simulink model "Three_phase_DAB_converter_2_"  (R2025b)
settings: Solver=VariableStepAuto  StartTime=0.0  StopTime=1  RelTol=1e-3
undefined symbols (not defined in the file): Ion, Lithium
libraries: eeRmsMeasurement x4, spsBatteryLib x2, spsUniversalBridgeLib x2, spsSeriesRLCBranchLib x2, eeGeneralControl x2, spsPower3phInstantaneousLib x2, spsThreePhaseVIMeasurementLib x2, spsThreePhaseSeriesRLCBranchLib x1, spsThreePhaseTransformerTwoWindingsLib x1, sps_lib x1
settings Model: Creator=91637  LastModifiedBy=DELL

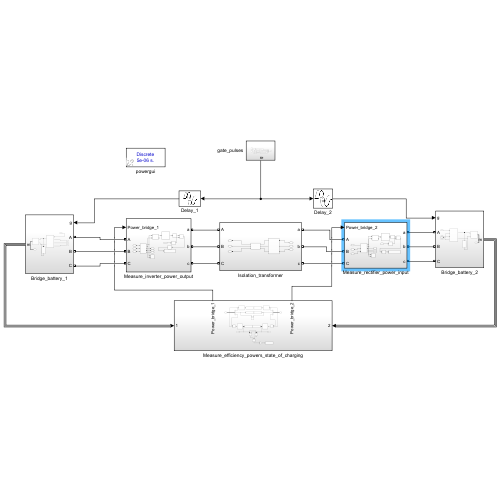
[thumbnail: Simulink's stored preview of the top-level diagram]
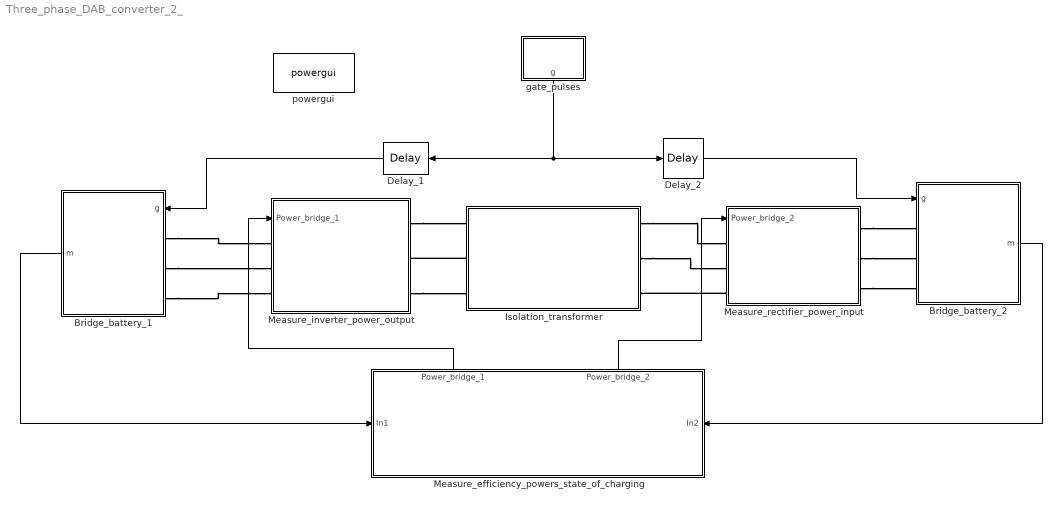
== system Three_phase_DAB_converter_2_ ==
  Bridge_battery_1 : Subsystem
  Bridge_battery_2 : Subsystem
  Delay_1 : TransportDelay  DelayTime=5e-6  BufferSize=1e5
  Delay_2 : TransportDelay  DelayTime=0
  Isolation_transformer : Subsystem
  Measure_efficiency_powers_state_of_charging : Subsystem
      settings: PortSchema="{\"entries\":[{\"content\":{\"sides\":[{\"content\":{\"connectorIds\":[\"In1\"]},\"type\":\"ConnectorPlacement.EquallySpacedRectSide\",\"uuid\":\"727947a8-7189-4754-ba39-ed4545685221\"},{\"content\":{\"connectorIds\":[\"In2\"],\"side\":\"RIGHT\"},\"type\":\"ConnectorPlacement.EquallySpacedRectSide\",\"uuid\":\"4f4ff040-aa02-42b0-ba60-9cf53e88cf93\"},{\"content\":{\"connectorIds\":[\"Out1\",\"Out2\"],\"side\":\"TOP\"},\"type\":\"ConnectorPlacement.EquallySpacedRectSide\",\"uuid\":\"ace19928-1506-4de9-a11d-c8770fc65bb2\"}]},\"type\":\"ConnectorPlacement.EquallySpacedConnector\",\"uuid\":\"7c6c4745-ab83-4df3-9031-3474db267f64\"}],\"packageUris\":[\"http://schema.mathworks.com/mf0/Connector/R2020b\"],\"version\":\"1.0\"}"
  Measure_inverter_power_output : Subsystem
  Measure_rectifier_power_input : Subsystem
  gate_pulses : Subsystem
  powergui : sps_lib/powergui  Priority=1  SimulationMode=Discrete  SampleTime=5e-6  frequency=60  Iterations=50  frequencyindice=0  Pbase=100e6  ErrMax=1e-4  UnitsV=kV  UnitsW=MW  buscounter=0  FunctionMessages=off  echomessages=off  EnableUseOfTLC=off  CurrentSourceSwitches=off  DisableSnubberDevices=off  DisableRonSwitches=off  DisableVfSwitches=off  DisplayEquations=off  AutomaticDiscreteSolvers=off  SolverType=Tustin/Backward Euler (TBE)  Interpol=off  ExternalGateDelay=off  methode=off  Ts=100  x0status=blocks  SPID=on  SwTol=0  HookPort=off  NonlinearTolerance=1e-4  nMaxIteration=100  ContinueOnMaxIteration=off  RestoreLinks=warning  ResistiveCurrentMeasurement=off  Frange=[0:2:500]  Ylog=off  Xlog=on  ShowGrid=off  save=off  variable=ZData  structure=0  ZoomFFT=off  StartTime=0.0  cycles=1  DisplayStyle=1  fundamental=60  FreqAxis=off  MaxFrequency=1000  frequencyindicesteady=1  RmsSteady=1  display=off
  wires:
  Bridge_battery_2/1(m) -> Measure_efficiency_powers_state_of_charging/2(In2)
  gate_pulses/1(g) -> Delay_2/1, Delay_1/1
  Bridge_battery_1/1(m) -> Measure_efficiency_powers_state_of_charging/1(In1)
  Measure_efficiency_powers_state_of_charging/2(Power_bridge_2) -> Measure_rectifier_power_input/1(Power_bridge_2)
  Measure_efficiency_powers_state_of_charging/1(Power_bridge_1) -> Measure_inverter_power_output/1(Power_bridge_1)
  Delay_1/1 -> Bridge_battery_1/1(g)
  Delay_2/1 -> Bridge_battery_2/1(g)
  connections:
  Isolation_transformer/RConn1 -- Measure_rectifier_power_input/LConn1
  Measure_rectifier_power_input/RConn1 -- Bridge_battery_2/LConn1
  Isolation_transformer/RConn2 -- Measure_rectifier_power_input/LConn2
  Measure_rectifier_power_input/RConn2 -- Bridge_battery_2/LConn2
  Measure_rectifier_power_input/LConn3 -- Isolation_transformer/RConn3
  Measure_rectifier_power_input/RConn3 -- Bridge_battery_2/LConn3
  Measure_inverter_power_output/RConn1 -- Isolation_transformer/LConn1
  Bridge_battery_1/LConn1 -- Measure_inverter_power_output/LConn1
  Isolation_transformer/LConn2 -- Measure_inverter_power_output/RConn2
  Bridge_battery_1/LConn2 -- Measure_inverter_power_output/LConn2
  Measure_inverter_power_output/RConn3 -- Isolation_transformer/LConn3
  Bridge_battery_1/LConn3 -- Measure_inverter_power_output/LConn3

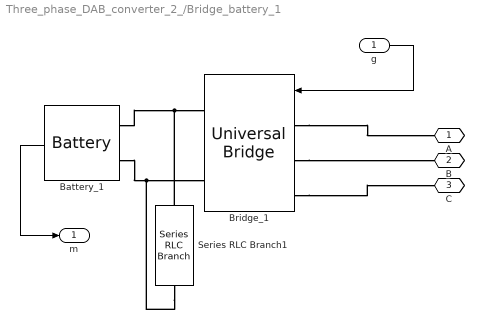
== system Three_phase_DAB_converter_2_/Bridge_battery_1 ==
  g : Inport
  Battery_1 : spsBatteryLib/Battery  BatType=Lithium-Ion  NomV=48  NomQ=20  SOC=80  Batt_Tr=0.01  PresetModel=on  MaxQ=20  MinV=36  FullV=55.8714  Dis_rate=8.6957  R=0.024  Normal_OP=18.087  expZone="[51.8585     0.982609]"
  Bridge_1 : spsUniversalBridgeLib/Universal Bridge  Arms=3  SnubberResistance=1e5  SnubberCapacitance=inf  Device=MOSFET / Diodes  Ron=1e-3  Lon=0  ForwardVoltages="[  0  0  ]"  ForwardVoltage=0  GTOparameters=[ 10e-6 , 20e-6 ]  IGBTparameters=[ 1e-6 , 2e-6 ]  Measurements=None  Measurements_2=None  converterType=Rectifier
      link override Status: GotoTag=T49_4813_4131163465740
  Series RLC Branch1 : spsSeriesRLCBranchLib/Series RLC Branch  LConnTagsString=__new0  RConnTagsString=__new0  BranchType=RC  Resistance=1000  Inductance=1e-3  SetiL0=off  InitialCurrent=0  Capacitance=1000e-6  Setx0=off  InitialVoltage=0  Measurements=None
  A : PMIOPort  Side=Left
  B : PMIOPort  Port=2  Side=Left
  C : PMIOPort  Port=3  Side=Left
  m : Outport
  wires:
  g/1 -> Bridge_1/1
  Battery_1/1 -> m/1
  connections:
  Bridge_1/LConn1 -- A/RConn1
  Battery_1/LConn2 -- Series RLC Branch1/RConn1 -- Bridge_1/RConn2
  Bridge_1/LConn3 -- C/RConn1
  Battery_1/LConn1 -- Series RLC Branch1/LConn1 -- Bridge_1/RConn1
  Bridge_1/LConn2 -- B/RConn1

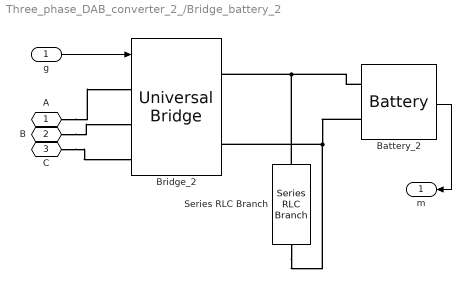
== system Three_phase_DAB_converter_2_/Bridge_battery_2 ==
  g : Inport
  Battery_2 : spsBatteryLib/Battery  BatType=Lithium-Ion  NomV=44  NomQ=20  SOC=40  Batt_Tr=0.01  PresetModel=on  MaxQ=20  MinV=33  FullV=51.2154  Dis_rate=8.6957  R=0.022  Normal_OP=18.087  expZone="[47.537     0.982609]"
  Bridge_2 : spsUniversalBridgeLib/Universal Bridge  Arms=3  SnubberResistance=1e5  SnubberCapacitance=inf  Device=MOSFET / Diodes  Ron=1e-3  Lon=0  ForwardVoltages="[  0  0  ]"  ForwardVoltage=0  GTOparameters=[ 10e-6 , 20e-6 ]  IGBTparameters=[ 1e-6 , 2e-6 ]  Measurements=None  Measurements_2=None  converterType=Rectifier
  Series RLC Branch : spsSeriesRLCBranchLib/Series RLC Branch  LConnTagsString=__new0  RConnTagsString=__new0  BranchType=RC  Resistance=1000  Inductance=1e-3  SetiL0=off  InitialCurrent=0  Capacitance=1000e-6  Setx0=off  InitialVoltage=0  Measurements=None
  A : PMIOPort  Side=Left
  B : PMIOPort  Port=2  Side=Left
  C : PMIOPort  Port=3  Side=Left
  m : Outport
  wires:
  g/1 -> Bridge_2/1
  Battery_2/1 -> m/1
  connections:
  C/RConn1 -- Bridge_2/LConn3
  Battery_2/LConn2 -- Series RLC Branch/RConn1 -- Bridge_2/RConn2
  B/RConn1 -- Bridge_2/LConn2
  Battery_2/LConn1 -- Bridge_2/RConn1 -- Series RLC Branch/LConn1
  A/RConn1 -- Bridge_2/LConn1

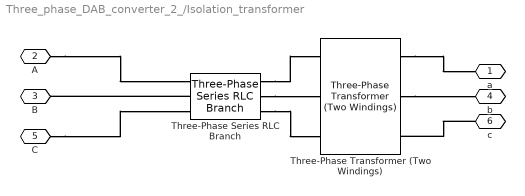
== system Three_phase_DAB_converter_2_/Isolation_transformer ==
  Three-Phase Series RLC Branch : spsThreePhaseSeriesRLCBranchLib/Three-Phase Series RLC Branch  LConnTagsString=A|B|C  RConnTagsString=A|B|C  BranchType=RL  Resistance=1e-2  Inductance=40e-6  Capacitance=1e-6  Measurements=None
  Three-Phase Transformer (Two Windings) : spsThreePhaseTransformerTwoWindingsLib/Three-Phase Transformer (Two Windings)  Winding1Connection=Yg  Winding2Connection=Yg  CoreType=Three single-phase transformers  SetSaturation=off  Hysteresis=off  DataFile='hysteresis'  SetInitialFlux=off  Measurements=None  UNITS=pu  NominalPower=[ 1e3 , 1e4 ]  Winding1=[230 0.003 0.01]  Winding2=[230 0.003 0.01]  Rm=500  Lm=200  L0=0.49999  Saturation=[0 0;0.0024 1.2;1 1.52]  InitialFluxes=[0.80001 -0.80001 0.7]  BreakLoop=off  DiscreteSolver=Trapezoidal iterative  DataType=off  TransfoNumber=1
  a : PMIOPort  Side=Right
  A : PMIOPort  Port=2  Side=Left
  B : PMIOPort  Port=3  Side=Left
  b : PMIOPort  Port=4  Side=Right
  C : PMIOPort  Port=5  Side=Left
  c : PMIOPort  Port=6  Side=Right
  connections:
  Three-Phase Series RLC Branch/RConn3 -- Three-Phase Transformer (Two Windings)/LConn3
  Three-Phase Transformer (Two Windings)/RConn1 -- a/RConn1
  c/RConn1 -- Three-Phase Transformer (Two Windings)/RConn3
  Three-Phase Transformer (Two Windings)/RConn2 -- b/RConn1
  Three-Phase Series RLC Branch/RConn1 -- Three-Phase Transformer (Two Windings)/LConn1
  A/RConn1 -- Three-Phase Series RLC Branch/LConn1
  Three-Phase Series RLC Branch/LConn2 -- B/RConn1
  Three-Phase Series RLC Branch/RConn2 -- Three-Phase Transformer (Two Windings)/LConn2
  C/RConn1 -- Three-Phase Series RLC Branch/LConn3

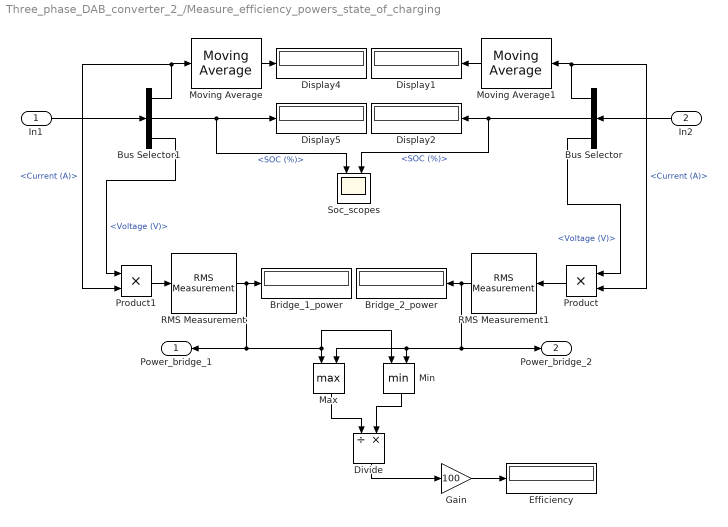
== system Three_phase_DAB_converter_2_/Measure_efficiency_powers_state_of_charging ==
  In1 : Inport
  In2 : Inport  Port=2
  Bridge_1_power : Display
  Bridge_2_power : Display
  Bus Selector : BusSelector  OutputSignals=Current (A),SOC (%),Voltage (V)
  Bus Selector1 : BusSelector  OutputSignals=Current (A),SOC (%),Voltage (V)
  Display{1..2,4..5} (4 alike) : Display
  Divide : Product  Inputs=/*
  Efficiency : Display
  Gain : Gain  Gain=100
  Max : MinMax  Function=max  Inputs=2
  Min : MinMax  Inputs=2
  Moving Average : eeGeneralControl/Moving Average  VariantControl=Variant1  LabelModeActiveChoice=Discrete  f=50  x0=0  BufferSize=8192  Ts=-1
      settings: LibrarySourceBlock=ee_sl_lib/General Control/Moving Average
  Moving Average1 : eeGeneralControl/Moving Average  VariantControl=Variant1  LabelModeActiveChoice=Discrete  f=50  x0=0  BufferSize=8192  Ts=-1
      settings: LibrarySourceBlock=ee_sl_lib/General Control/Moving Average
  Product : Product
  Product1 : Product
  RMS Measurement : eeRmsMeasurement/RMS Measurement  LabelModeActiveChoice=Total  F=60  SpecifyHarmonics=off  K=[0 1 2]  Ts=0
      settings: LibrarySourceBlock=|
      | ee_sl_lib/Measurements/RMS
      | Measurement
  RMS Measurement1 : eeRmsMeasurement/RMS Measurement  LabelModeActiveChoice=Total  F=60  SpecifyHarmonics=off  K=[0 1 2]  Ts=0
      settings: LibrarySourceBlock=|
      | ee_sl_lib/Measurements/RMS
      | Measurement
  Soc_scopes : Scope  NumInputPorts=2
      settings: ActiveDisplayYMinimum=80.6573374913129  ActiveDisplayYMaximum=80.660364899071055  DataLoggingVariableName=ScopeData2
  Power_bridge_1 : Outport  VectorParamsAs1DForOutWhenUnconnected=off
  Power_bridge_2 : Outport  Port=2
  wires:
  Product1/1 -> RMS Measurement/1
  Bus Selector1/1 -> Product1/2, Moving Average/1  "<Current (A)>"
  RMS Measurement1/1 -> Min/2, Max/2, Power_bridge_2/1, Bridge_2_power/1
  Bus Selector/1 -> Moving Average1/1, Product/2  "<Current (A)>"
  Moving Average1/1 -> Display1/1
  Bus Selector1/2 -> Soc_scopes/1, Display5/1  "<SOC (%)>"
  Bus Selector1/3 -> Product1/1  "<Voltage (V)>"
  Bus Selector/2 -> Soc_scopes/2, Display2/1  "<SOC (%)>"
  Moving Average/1 -> Display4/1
  In1/1 -> Bus Selector1/1
  Bus Selector/3 -> Product/1  "<Voltage (V)>"
  Product/1 -> RMS Measurement1/1
  RMS Measurement/1 -> Min/1, Max/1, Power_bridge_1/1, Bridge_1_power/1
  In2/1 -> Bus Selector/1
  Divide/1 -> Gain/1
  Gain/1 -> Efficiency/1
  Max/1 -> Divide/1
  Min/1 -> Divide/2

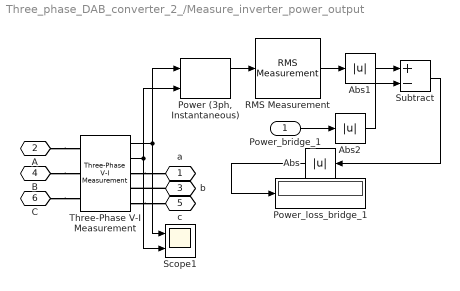
== system Three_phase_DAB_converter_2_/Measure_inverter_power_output ==
  Power_bridge_1 : Inport
  Abs : Abs  SaturateOnIntegerOverflow=off
  Abs1 : Abs  SaturateOnIntegerOverflow=off
  Abs2 : Abs  SaturateOnIntegerOverflow=off
  "Power (3ph, Instantaneous)" : spsPower3phInstantaneousLib/Power (3ph, Instantaneous)
  Power_loss_bridge_1 : Display
  RMS Measurement : eeRmsMeasurement/RMS Measurement  LabelModeActiveChoice=Total  F=60  SpecifyHarmonics=off  K=[0 1 2]  Ts=0
      settings: LibrarySourceBlock=|
      | ee_sl_lib/Measurements/RMS
      | Measurement
  Scope1 : Scope  NumInputPorts=2
      settings: ActiveDisplayYMinimum=-87.331585407459983  ActiveDisplayYMaximum=86.18489489271434
  Subtract : Sum  Inputs=+-
  Three-Phase V-I Measurement : spsThreePhaseVIMeasurementLib/Three-Phase V-I Measurement  VoltageMeasurement=phase-to-ground  SetLabelV=off  LabelV=Vabc  Vpu=off  VpuLL=off  CurrentMeasurement=yes  SetLabelI=off  LabelI=Iabc  Ipu=off  Pbase=100e6  Vbase=500e3  OutputType=Complex  PhasorSimulation=off  PSBequivalent=0
  a : PMIOPort  Side=Right
  A : PMIOPort  Port=2  Side=Left
  b : PMIOPort  Port=3  Side=Right
  B : PMIOPort  Port=4  Side=Left
  c : PMIOPort  Port=5  Side=Right
  C : PMIOPort  Port=6  Side=Left
  wires:
  Three-Phase V-I Measurement/1 -> "Power (3ph, Instantaneous)"/1, Scope1/1
  Three-Phase V-I Measurement/2 -> "Power (3ph, Instantaneous)"/2, Scope1/2
  "Power (3ph, Instantaneous)"/1 -> RMS Measurement/1
  Abs/1 -> Power_loss_bridge_1/1
  Subtract/1 -> Abs/1
  Power_bridge_1/1 -> Abs2/1
  RMS Measurement/1 -> Abs1/1
  Abs1/1 -> Subtract/1
  Abs2/1 -> Subtract/2
  connections:
  b/RConn1 -- Three-Phase V-I Measurement/RConn2
  Three-Phase V-I Measurement/RConn3 -- c/RConn1
  Three-Phase V-I Measurement/RConn1 -- a/RConn1
  A/RConn1 -- Three-Phase V-I Measurement/LConn1
  B/RConn1 -- Three-Phase V-I Measurement/LConn2
  C/RConn1 -- Three-Phase V-I Measurement/LConn3

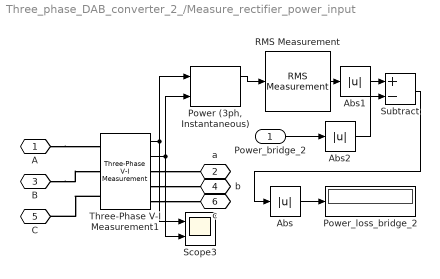
== system Three_phase_DAB_converter_2_/Measure_rectifier_power_input ==
  Power_bridge_2 : Inport
  Abs : Abs  SaturateOnIntegerOverflow=off
  Abs1 : Abs  SaturateOnIntegerOverflow=off
  Abs2 : Abs  SaturateOnIntegerOverflow=off
  "Power (3ph, Instantaneous)" : spsPower3phInstantaneousLib/Power (3ph, Instantaneous)
  Power_loss_bridge_2 : Display
  RMS Measurement : eeRmsMeasurement/RMS Measurement  LabelModeActiveChoice=Total  F=60  SpecifyHarmonics=off  K=[0 1 2]  Ts=0
      settings: LibrarySourceBlock=|
      | ee_sl_lib/Measurements/RMS
      | Measurement
  Scope3 : Scope  NumInputPorts=2
      settings: ActiveDisplayYMinimum=-87.331585407459983  ActiveDisplayYMaximum=86.18489489271434  DataLoggingVariableName=ScopeData3
  Subtract : Sum  Inputs=+-
  Three-Phase V-I Measurement1 : spsThreePhaseVIMeasurementLib/Three-Phase V-I Measurement  VoltageMeasurement=phase-to-ground  SetLabelV=off  LabelV=Vabc  Vpu=off  VpuLL=off  CurrentMeasurement=yes  SetLabelI=off  LabelI=Iabc  Ipu=off  Pbase=100e6  Vbase=500e3  OutputType=Complex  PhasorSimulation=off  PSBequivalent=0
  A : PMIOPort  Side=Left
  a : PMIOPort  Port=2  Side=Right
  B : PMIOPort  Port=3  Side=Left
  b : PMIOPort  Port=4  Side=Right
  C : PMIOPort  Port=5  Side=Left
  c : PMIOPort  Port=6  Side=Right
  wires:
  Three-Phase V-I Measurement1/1 -> "Power (3ph, Instantaneous)"/1, Scope3/1
  Three-Phase V-I Measurement1/2 -> "Power (3ph, Instantaneous)"/2, Scope3/2
  "Power (3ph, Instantaneous)"/1 -> RMS Measurement/1
  Power_bridge_2/1 -> Abs2/1
  Subtract/1 -> Abs/1
  Abs/1 -> Power_loss_bridge_2/1
  RMS Measurement/1 -> Abs1/1
  Abs1/1 -> Subtract/1
  Abs2/1 -> Subtract/2
  connections:
  Three-Phase V-I Measurement1/RConn2 -- b/RConn1
  B/RConn1 -- Three-Phase V-I Measurement1/LConn2
  Three-Phase V-I Measurement1/LConn3 -- C/RConn1
  Three-Phase V-I Measurement1/RConn3 -- c/RConn1
  A/RConn1 -- Three-Phase V-I Measurement1/LConn1
  Three-Phase V-I Measurement1/RConn1 -- a/RConn1

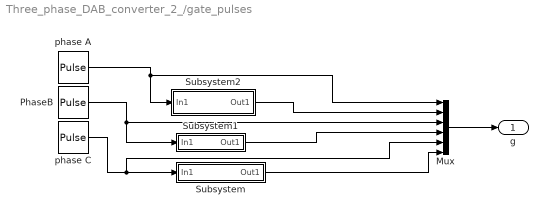
== system Three_phase_DAB_converter_2_/gate_pulses ==
  " PhaseB" : DiscretePulseGenerator  PulseType=Time based  Period=5e-5  PulseWidth=50  PhaseDelay=(5e-5)/3
  " phase C" : DiscretePulseGenerator  PulseType=Time based  Period=5e-5  PulseWidth=50  PhaseDelay=-(5e-5)/3
  Mux : Mux  Inputs=6
  Subsystem : Subsystem
  Subsystem1 : Subsystem
  Subsystem2 : Subsystem
  phase A : DiscretePulseGenerator  PulseType=Time based  Period=5e-5  PulseWidth=50
  g : Outport
  wires:
  " phase C"/1 -> Subsystem/1(In1), Mux/5
  Subsystem1/1(Out1) -> Mux/4
  " PhaseB"/1 -> Subsystem1/1(In1), Mux/3
  phase A/1 -> Subsystem2/1(In1), Mux/1
  Subsystem/1(Out1) -> Mux/6
  Subsystem2/1(Out1) -> Mux/2
  Mux/1 -> g/1

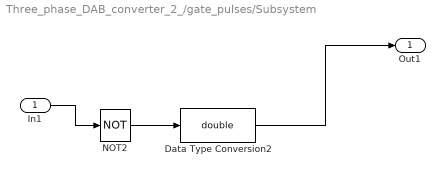
== system Three_phase_DAB_converter_2_/gate_pulses/Subsystem ==
  In1 : Inport
  Data Type Conversion2 : DataTypeConversion  OutDataTypeStr=double  SaturateOnIntegerOverflow=off  RndMeth=Floor
  NOT2 : Logic  Operator=NOT  IconShape=distinctive  AllPortsSameDT=off  OutDataTypeStr=boolean
  Out1 : Outport
  wires:
  Data Type Conversion2/1 -> Out1/1
  NOT2/1 -> Data Type Conversion2/1
  In1/1 -> NOT2/1

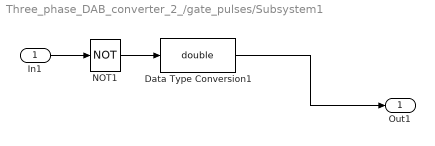
== system Three_phase_DAB_converter_2_/gate_pulses/Subsystem1 ==
  In1 : Inport
  Data Type Conversion1 : DataTypeConversion  OutDataTypeStr=double  SaturateOnIntegerOverflow=off  RndMeth=Floor
  NOT1 : Logic  Operator=NOT  IconShape=distinctive  AllPortsSameDT=off  OutDataTypeStr=boolean
  Out1 : Outport
  wires:
  NOT1/1 -> Data Type Conversion1/1
  In1/1 -> NOT1/1
  Data Type Conversion1/1 -> Out1/1

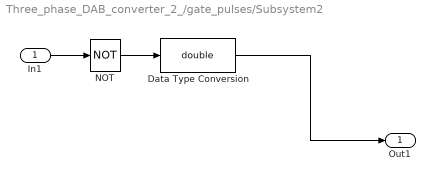
== system Three_phase_DAB_converter_2_/gate_pulses/Subsystem2 ==
  In1 : Inport
  Data Type Conversion : DataTypeConversion  OutDataTypeStr=double  SaturateOnIntegerOverflow=off  RndMeth=Floor
  NOT : Logic  Operator=NOT  IconShape=distinctive  AllPortsSameDT=off  OutDataTypeStr=boolean
  Out1 : Outport
  wires:
  NOT/1 -> Data Type Conversion/1
  In1/1 -> NOT/1
  Data Type Conversion/1 -> Out1/1
